simulink model "s_cd_hmc_reord_build_ramp"  (R2016b)
settings: Solver=VariableStepAuto  StartTime=0.0  StopTime=1000  RelTol=1e-3  EnableMultiTasking=on
undefined symbols (not defined in the file): Down, fft_stages, Up
libraries: xbsIndex_r4 x4695, casper_library_misc x3
(part 7 of 31)

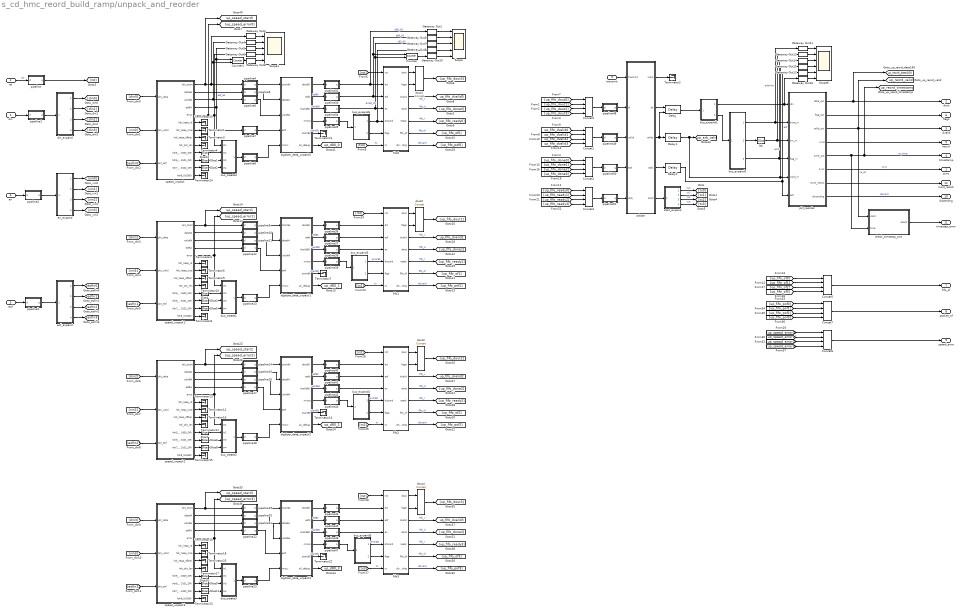
== system s_cd_hmc_reord_build_ramp/unpack_and_reorder ==
  rst : Inport
  din : Inport  Port=2
  eof : Inport  Port=3
  en : Inport  Port=4
  transmit : Inport  Port=5
  Concat{1..7} (7 alike) : xbsIndex_r4/Concat  num_inputs=4  dbl_ovrd=off  block_type=concat
  Counter : xbsIndex_r4/Counter  cnt_type=Free Running  cnt_to=Inf  operation=Up  start_count=0  cnt_by_val=1  arith_type=Unsigned  n_bits=10  bin_pt=0  load_pin=off  rst=on  en=on  explicit_period=on  period=1  use_behavioral_HDL=on  implementation=Fabric  dbl_ovrd=off  block_type=counter
  Counter1 : xbsIndex_r4/Counter  cnt_type=Free Running  cnt_to=Inf  operation=Up  start_count=0  cnt_by_val=1  arith_type=Unsigned  n_bits=10  bin_pt=0  load_pin=off  rst=on  en=on  explicit_period=on  period=1  use_behavioral_HDL=on  implementation=Fabric  dbl_ovrd=off  block_type=counter
  Delay : xbsIndex_r4/Delay  rst=off  infoeditControl=Selection of Reset will increase slice count due to use of real FFs and instead of SRLs  en=on  latency=1  reg_retiming=on  dbl_ovrd=off  block_type=delay
  Delay1 : xbsIndex_r4/Delay  rst=off  infoeditControl=Selection of Reset will increase slice count due to use of real FFs and instead of SRLs  en=off  latency=1  reg_retiming=on  dbl_ovrd=off  block_type=delay
  Delay2 : xbsIndex_r4/Delay  rst=off  infoeditControl=Selection of Reset will increase slice count due to use of real FFs and instead of SRLs  en=off  latency=1  reg_retiming=on  dbl_ovrd=off  block_type=delay
  Gateway Out{1..16} (16 alike) : xbsIndex_r4/Gateway Out  inherit_from_input=off  hdl_port=off  rows=1  columns=1  UseAsDAC=off  DACChannel='1'  interface=None  automatic_assignment=on  address_offset=hex2dec('00')  intf_name=''  intf_description=''  timing_constraint=None  locs_specified=off  LOCs={}  io_standard={}  block_type=gatewayout
  Scope : Scope  NumInputPorts=5
  Scope1 : Scope  NumInputPorts=5
  Scope6 : Scope  NumInputPorts=6
  Slice{1..3,5..6,8..9,11} (8 alike) : xbsIndex_r4/Slice  nbits=2  boolean_output=off  mode=Lower Bit Location + Width  bit1=0  base1=MSB of Input  bit0=0  base0=LSB of Input  dbl_ovrd=off  block_type=slice
  Slice{4,7,10,12} (4 alike) : xbsIndex_r4/Slice  nbits=48 - n_bits_timestep  boolean_output=off  mode=Upper Bit Location + Width  bit1=0  base1=MSB of Input  bit0=0  base0=LSB of Input  dbl_ovrd=off  block_type=slice
  Terminator{1..25} (25 alike) : Terminator
  arbiter : Subsystem  mask{n_inputs=4, n_bits_input=160 + 48 - n_bits_timestep + 2 + 2, mux_latency=2}
      mask prompts: n_inputs "number of inputs"; n_bits_input "input bit widths"; mux_latency "mux latency"
      mask init:
      | set_param([gcb, '/eofi_mux'], ...
      |     'n_bits', 'ones(1, n_inputs)', ...
      |     'mux_latency', 'mux_latency', ...
      |     'cmplx', 'off', 'misc', 'off');
      | set_param([gcb, '/di_mux'], ...
      |     'n_bits', 'repmat(n_bits_input, 1, n_inputs)', ...
      |     'mux_latency', 'mux_latency', ...
      |     'cmplx', 'off', 'misc', 'off');
      | set_param([gcb, '/validi_mux'], ...
      |     'n_bits', 'ones(1, n_inputs)', ...
      |     'mux_latency', 'mux_latency', ...
      |     'cmplx', 'off', 'misc', 'off');
      | set_param([gcb, '/busy_edge_rep'], ...
      |     'replication', 'n_inputs', ...
      |     'misc', 'off');
  bus_create1 : Subsystem  AncestorBlock=casper_library_flow_control/bus_create  mask(bus_create){inputNum=4}
      mask prompts: inputNum "Number of inputs:"
      mask init:
      | bus_create_init(gcb,...
      |     'inputNum', inputNum);
  bus_create2 : Subsystem  AncestorBlock=casper_library_flow_control/bus_create  mask(bus_create){inputNum=4}
      mask prompts: inputNum "Number of inputs:"
      mask init:
      | bus_create_init(gcb,...
      |     'inputNum', inputNum);
  bus_create3 : Subsystem  AncestorBlock=casper_library_flow_control/bus_create  mask(bus_create){inputNum=4}
      mask prompts: inputNum "Number of inputs:"
      mask init:
      | bus_create_init(gcb,...
      |     'inputNum', inputNum);
  bus_create4 : Subsystem  AncestorBlock=casper_library_flow_control/bus_create  mask(bus_create){inputNum=4}
      mask prompts: inputNum "Number of inputs:"
      mask init:
      | bus_create_init(gcb,...
      |     'inputNum', inputNum);
  bus_expand1 : Subsystem  AncestorBlock=casper_library_flow_control/bus_expand  mask(bus_expand){mode=divisions of arbitrary size, outputNum=1, outputWidth=[160, sum([48 - n_bits_timestep, 2, 2])], outputBinaryPt=[0 0], outputArithmeticType=[0 0], show_format=off, outputToWorkspace=off, variablePrefix=out, outputToModelAsWell=on}
      mask prompts: outputNum "Number of outputs:"; outputWidth "Output width [msb ... lsb]:"; outputBinaryPt "Output binary point position [msb ... lsb]:"; outputArithmeticType "Output arithmetic type (ufix=0, fix=1, bool=2) [msb ... lsb]:"; show_format "Print format string?"; outputToWorkspace "Output to workspace?"; variablePrefix "Variable name prefix:"; outputToModelAsWell "Output to model as well?"
      mask help:
      | Expands a 'bus' made using a bus_create or Xilinx
      | concat block.
      | The input will be divided into the specified number
      | of outputs with the specified arithmetic types.
      | Divisions are made from most significant bit.
      mask init: same as s_cd_hmc_reord_build_ramp/bus_expand
      settings: AttributesFormatString=2 outputs
      mask TypeOptions mode: divisions of equal size | divisions of arbitrary size
      mask Callback mode: bus_expand_callback();
      mask Callback outputWidth: bus_expand_callback();
      mask Callback outputToWorkspace: bus_expand_callback();
  bus_expand2 : Subsystem  AncestorBlock=casper_library_flow_control/bus_expand  mask(bus_expand){mode=divisions of arbitrary size, outputNum=1, outputWidth=[48 - n_bits_timestep, 2, 2], outputBinaryPt=[0 0 0], outputArithmeticType=[0 0 0], show_format=off, outputToWorkspace=off, variablePrefix=out, outputToModelAsWell=on}
      mask prompts: outputNum "Number of outputs:"; outputWidth "Output width [msb ... lsb]:"; outputBinaryPt "Output binary point position [msb ... lsb]:"; outputArithmeticType "Output arithmetic type (ufix=0, fix=1, bool=2) [msb ... lsb]:"; show_format "Print format string?"; outputToWorkspace "Output to workspace?"; variablePrefix "Variable name prefix:"; outputToModelAsWell "Output to model as well?"
      mask help:
      | Expands a 'bus' made using a bus_create or Xilinx
      | concat block.
      | The input will be divided into the specified number
      | of outputs with the specified arithmetic types.
      | Divisions are made from most significant bit.
      mask init: same as s_cd_hmc_reord_build_ramp/bus_expand
      settings: AttributesFormatString=3 outputs
      mask TypeOptions mode: divisions of equal size | divisions of arbitrary size
      mask Callback mode: bus_expand_callback();
      mask Callback outputWidth: bus_expand_callback();
      mask Callback outputToWorkspace: bus_expand_callback();
  bus_expand3 : Subsystem  AncestorBlock=casper_library_flow_control/bus_expand  mask(bus_expand){mode=divisions of arbitrary size, outputNum=1, outputWidth=[1, sum([48 - n_bits_timestep, 2, 2])], outputBinaryPt=[0 0], outputArithmeticType=[2 0], show_format=off, outputToWorkspace=off, variablePrefix=out, outputToModelAsWell=on}
      mask prompts: outputNum "Number of outputs:"; outputWidth "Output width [msb ... lsb]:"; outputBinaryPt "Output binary point position [msb ... lsb]:"; outputArithmeticType "Output arithmetic type (ufix=0, fix=1, bool=2) [msb ... lsb]:"; show_format "Print format string?"; outputToWorkspace "Output to workspace?"; variablePrefix "Variable name prefix:"; outputToModelAsWell "Output to model as well?"
      mask help:
      | Expands a 'bus' made using a bus_create or Xilinx
      | concat block.
      | The input will be divided into the specified number
      | of outputs with the specified arithmetic types.
      | Divisions are made from most significant bit.
      mask init: same as s_cd_hmc_reord_build_ramp/bus_expand
      settings: AttributesFormatString=2 outputs
      mask TypeOptions mode: divisions of equal size | divisions of arbitrary size
      mask Callback mode: bus_expand_callback();
      mask Callback outputWidth: bus_expand_callback();
      mask Callback outputToWorkspace: bus_expand_callback();
  bus_expand4 : Subsystem  AncestorBlock=casper_library_flow_control/bus_expand  mask(bus_expand){mode=divisions of arbitrary size, outputNum=1, outputWidth=[1, sum([48 - n_bits_timestep, 2, 2])], outputBinaryPt=[0 0], outputArithmeticType=[2 0], show_format=off, outputToWorkspace=off, variablePrefix=out, outputToModelAsWell=on}
      mask prompts: outputNum "Number of outputs:"; outputWidth "Output width [msb ... lsb]:"; outputBinaryPt "Output binary point position [msb ... lsb]:"; outputArithmeticType "Output arithmetic type (ufix=0, fix=1, bool=2) [msb ... lsb]:"; show_format "Print format string?"; outputToWorkspace "Output to workspace?"; variablePrefix "Variable name prefix:"; outputToModelAsWell "Output to model as well?"
      mask help:
      | Expands a 'bus' made using a bus_create or Xilinx
      | concat block.
      | The input will be divided into the specified number
      | of outputs with the specified arithmetic types.
      | Divisions are made from most significant bit.
      mask init: same as s_cd_hmc_reord_build_ramp/bus_expand
      settings: AttributesFormatString=2 outputs
      mask TypeOptions mode: divisions of equal size | divisions of arbitrary size
      mask Callback mode: bus_expand_callback();
      mask Callback outputWidth: bus_expand_callback();
      mask Callback outputToWorkspace: bus_expand_callback();
  bus_expand5 : Subsystem  AncestorBlock=casper_library_flow_control/bus_expand  mask(bus_expand){mode=divisions of arbitrary size, outputNum=1, outputWidth=[1, sum([48 - n_bits_timestep, 2, 2])], outputBinaryPt=[0 0], outputArithmeticType=[2 0], show_format=off, outputToWorkspace=off, variablePrefix=out, outputToModelAsWell=on}
      mask prompts: outputNum "Number of outputs:"; outputWidth "Output width [msb ... lsb]:"; outputBinaryPt "Output binary point position [msb ... lsb]:"; outputArithmeticType "Output arithmetic type (ufix=0, fix=1, bool=2) [msb ... lsb]:"; show_format "Print format string?"; outputToWorkspace "Output to workspace?"; variablePrefix "Variable name prefix:"; outputToModelAsWell "Output to model as well?"
      mask help:
      | Expands a 'bus' made using a bus_create or Xilinx
      | concat block.
      | The input will be divided into the specified number
      | of outputs with the specified arithmetic types.
      | Divisions are made from most significant bit.
      mask init: same as s_cd_hmc_reord_build_ramp/bus_expand
      settings: AttributesFormatString=2 outputs
      mask TypeOptions mode: divisions of equal size | divisions of arbitrary size
      mask Callback mode: bus_expand_callback();
      mask Callback outputWidth: bus_expand_callback();
      mask Callback outputToWorkspace: bus_expand_callback();
  bus_expand6 : Subsystem  AncestorBlock=casper_library_flow_control/bus_expand  mask(bus_expand){mode=divisions of arbitrary size, outputNum=1, outputWidth=[1, sum([48 - n_bits_timestep, 2, 2])], outputBinaryPt=[0 0], outputArithmeticType=[2 0], show_format=off, outputToWorkspace=off, variablePrefix=out, outputToModelAsWell=on}
      mask prompts: outputNum "Number of outputs:"; outputWidth "Output width [msb ... lsb]:"; outputBinaryPt "Output binary point position [msb ... lsb]:"; outputArithmeticType "Output arithmetic type (ufix=0, fix=1, bool=2) [msb ... lsb]:"; show_format "Print format string?"; outputToWorkspace "Output to workspace?"; variablePrefix "Variable name prefix:"; outputToModelAsWell "Output to model as well?"
      mask help:
      | Expands a 'bus' made using a bus_create or Xilinx
      | concat block.
      | The input will be divided into the specified number
      | of outputs with the specified arithmetic types.
      | Divisions are made from most significant bit.
      mask init: same as s_cd_hmc_reord_build_ramp/bus_expand
      settings: AttributesFormatString=2 outputs
      mask TypeOptions mode: divisions of equal size | divisions of arbitrary size
      mask Callback mode: bus_expand_callback();
      mask Callback outputWidth: bus_expand_callback();
      mask Callback outputToWorkspace: bus_expand_callback();
  check_timestep_one : Subsystem
  digitiser_data_unpack0 : Subsystem
  digitiser_data_unpack1 : Subsystem
  digitiser_data_unpack2 : Subsystem
  digitiser_data_unpack3 : Subsystem
  din_expand : Subsystem  AncestorBlock=casper_library_flow_control/bus_expand  mask(bus_expand){mode=divisions of equal size, outputNum=4, outputWidth=64, outputBinaryPt=0, outputArithmeticType=0, show_format=off, outputToWorkspace=off, variablePrefix=out, outputToModelAsWell=on}
      mask prompts: outputNum "Number of outputs:"; outputWidth "Output width:"; outputBinaryPt "Output binary point position:"; outputArithmeticType "Output arithmetic type (ufix=0, fix=1, bool=2):"; show_format "Print format string?"; outputToWorkspace "Output to workspace?"; variablePrefix "Variable name prefix:"; outputToModelAsWell "Output to model as well?"
      mask help:
      | Expands a 'bus' made using a bus_create or Xilinx
      | concat block.
      | The input will be divided into the specified number
      | of outputs with the specified arithmetic types.
      | Divisions are made from most significant bit.
      mask init: same as s_cd_hmc_reord_build_ramp/bus_expand
      settings: AttributesFormatString=4 outputs
      mask TypeOptions mode: divisions of equal size | divisions of arbitrary size
      mask Callback mode: bus_expand_callback();
      mask Callback outputWidth: bus_expand_callback();
      mask Callback outputToWorkspace: bus_expand_callback();
  dout{1..4} (4 alike) : xbsIndex_r4/Concat  num_inputs=2  dbl_ovrd=off  block_type=concat
  en_expand : Subsystem  AncestorBlock=casper_library_flow_control/bus_expand  mask(bus_expand){mode=divisions of equal size, outputNum=4, outputWidth=1, outputBinaryPt=0, outputArithmeticType=2, show_format=off, outputToWorkspace=off, variablePrefix=out, outputToModelAsWell=on}
      mask prompts: outputNum "Number of outputs:"; outputWidth "Output width:"; outputBinaryPt "Output binary point position:"; outputArithmeticType "Output arithmetic type (ufix=0, fix=1, bool=2):"; show_format "Print format string?"; outputToWorkspace "Output to workspace?"; variablePrefix "Variable name prefix:"; outputToModelAsWell "Output to model as well?"
      mask help:
      | Expands a 'bus' made using a bus_create or Xilinx
      | concat block.
      | The input will be divided into the specified number
      | of outputs with the specified arithmetic types.
      | Divisions are made from most significant bit.
      mask init: same as s_cd_hmc_reord_build_ramp/bus_expand
      settings: AttributesFormatString=4 outputs
      mask TypeOptions mode: divisions of equal size | divisions of arbitrary size
      mask Callback mode: bus_expand_callback();
      mask Callback outputWidth: bus_expand_callback();
      mask Callback outputToWorkspace: bus_expand_callback();
  eof_expand : Subsystem  AncestorBlock=casper_library_flow_control/bus_expand  mask(bus_expand){mode=divisions of equal size, outputNum=4, outputWidth=1, outputBinaryPt=0, outputArithmeticType=2, show_format=off, outputToWorkspace=off, variablePrefix=out, outputToModelAsWell=on}
      mask prompts: outputNum "Number of outputs:"; outputWidth "Output width:"; outputBinaryPt "Output binary point position:"; outputArithmeticType "Output arithmetic type (ufix=0, fix=1, bool=2):"; show_format "Print format string?"; outputToWorkspace "Output to workspace?"; variablePrefix "Variable name prefix:"; outputToModelAsWell "Output to model as well?"
      mask help:
      | Expands a 'bus' made using a bus_create or Xilinx
      | concat block.
      | The input will be divided into the specified number
      | of outputs with the specified arithmetic types.
      | Divisions are made from most significant bit.
      mask init: same as s_cd_hmc_reord_build_ramp/bus_expand
      settings: AttributesFormatString=4 outputs
      mask TypeOptions mode: divisions of equal size | divisions of arbitrary size
      mask Callback mode: bus_expand_callback();
      mask Callback outputWidth: bus_expand_callback();
      mask Callback outputToWorkspace: bus_expand_callback();
  fifo0 : Subsystem  mask{n_bits_din=80, scale_factor_bits=1, input_word_count_bits=n_bits_packet_size, n_bits_depth=n_bits_fifo_depth, n_bits_flag=sum([48 - n_bits_timestep, 2, 2]), bram_latency=bram_latency}
      mask prompts: n_bits_din "input data bit width"; scale_factor_bits "output width scale factor (2^? input bits)"; input_word_count_bits "max input word count (2^?)"; n_bits_depth "max buffer depth (2^? packets)"; n_bits_flag "flag bit width"; bram_latency "BRAM latency"
  fifo1 : Subsystem  mask{n_bits_din=80, scale_factor_bits=1, input_word_count_bits=n_bits_packet_size, n_bits_depth=n_bits_fifo_depth, n_bits_flag=sum([48 - n_bits_timestep, 2, 2]), bram_latency=bram_latency}
      mask prompts: n_bits_din "input data bit width"; scale_factor_bits "output width scale factor (2^? input bits)"; input_word_count_bits "max input word count (2^?)"; n_bits_depth "max buffer depth (2^? packets)"; n_bits_flag "flag bit width"; bram_latency "BRAM latency"
  fifo2 : Subsystem  mask{n_bits_din=80, scale_factor_bits=1, input_word_count_bits=n_bits_packet_size, n_bits_depth=n_bits_fifo_depth, n_bits_flag=sum([48 - n_bits_timestep, 2, 2]), bram_latency=bram_latency}
      mask prompts: n_bits_din "input data bit width"; scale_factor_bits "output width scale factor (2^? input bits)"; input_word_count_bits "max input word count (2^?)"; n_bits_depth "max buffer depth (2^? packets)"; n_bits_flag "flag bit width"; bram_latency "BRAM latency"
  fifo3 : Subsystem  mask{n_bits_din=80, scale_factor_bits=1, input_word_count_bits=n_bits_packet_size, n_bits_depth=n_bits_fifo_depth, n_bits_flag=sum([48 - n_bits_timestep, 2, 2]), bram_latency=bram_latency}
      mask prompts: n_bits_din "input data bit width"; scale_factor_bits "output width scale factor (2^? input bits)"; input_word_count_bits "max input word count (2^?)"; n_bits_depth "max buffer depth (2^? packets)"; n_bits_flag "flag bit width"; bram_latency "BRAM latency"
  lsb : xbsIndex_r4/Slice  nbits=1  boolean_output=off  mode=Lower Bit Location + Width  bit1=0  base1=MSB of Input  bit0=0  base0=LSB of Input  dbl_ovrd=off  block_type=slice
  pipeline : Subsystem  AncestorBlock=casper_library_delays/pipeline  mask(pipeline){latency=2}
      mask help:
      | An explicitly laid-out delay line to avoid mapping to SRL16s
      | for use in pipelining to help achieve timing closure.
      mask init:
      | pipeline_init(gcb,'latency',latency);
      settings: AttributesFormatString=Latency = %<latency>
      mask Display:
      | port_label('input', 1, 'd');
      | port_label('output', 1, 'q');
      | disp(['Z^-', num2str(latency)]);
  pipeline1 : Subsystem  AncestorBlock=casper_library_delays/pipeline  mask(pipeline){latency=2}
      mask help:
      | An explicitly laid-out delay line to avoid mapping to SRL16s
      | for use in pipelining to help achieve timing closure.
      mask init:
      | pipeline_init(gcb,'latency',latency);
      settings: AttributesFormatString=Latency = %<latency>
      mask Display:
      | port_label('input', 1, 'd');
      | port_label('output', 1, 'q');
      | disp(['Z^-', num2str(latency)]);
  pipeline10 : Subsystem  AncestorBlock=casper_library_delays/pipeline  mask(pipeline){latency=2}
      mask help:
      | An explicitly laid-out delay line to avoid mapping to SRL16s
      | for use in pipelining to help achieve timing closure.
      mask init:
      | pipeline_init(gcb,'latency',latency);
      settings: AttributesFormatString=Latency = %<latency>
      mask Display:
      | port_label('input', 1, 'd');
      | port_label('output', 1, 'q');
      | disp(['Z^-', num2str(latency)]);
  pipeline11 : Subsystem  AncestorBlock=casper_library_delays/pipeline  mask(pipeline){latency=2}
      mask help:
      | An explicitly laid-out delay line to avoid mapping to SRL16s
      | for use in pipelining to help achieve timing closure.
      mask init:
      | pipeline_init(gcb,'latency',latency);
      settings: AttributesFormatString=Latency = %<latency>
      mask Display:
      | port_label('input', 1, 'd');
      | port_label('output', 1, 'q');
      | disp(['Z^-', num2str(latency)]);
  pipeline12 : Subsystem  AncestorBlock=casper_library_delays/pipeline  mask(pipeline){latency=2}
      mask help:
      | An explicitly laid-out delay line to avoid mapping to SRL16s
      | for use in pipelining to help achieve timing closure.
      mask init:
      | pipeline_init(gcb,'latency',latency);
      settings: AttributesFormatString=Latency = %<latency>
      mask Display:
      | port_label('input', 1, 'd');
      | port_label('output', 1, 'q');
      | disp(['Z^-', num2str(latency)]);
  pipeline13 : Subsystem  AncestorBlock=casper_library_delays/pipeline  mask(pipeline){latency=2}
      mask help:
      | An explicitly laid-out delay line to avoid mapping to SRL16s
      | for use in pipelining to help achieve timing closure.
      mask init:
      | pipeline_init(gcb,'latency',latency);
      settings: AttributesFormatString=Latency = %<latency>
      mask Display:
      | port_label('input', 1, 'd');
      | port_label('output', 1, 'q');
      | disp(['Z^-', num2str(latency)]);
  pipeline14 : Subsystem  AncestorBlock=casper_library_delays/pipeline  mask(pipeline){latency=2}
      mask help:
      | An explicitly laid-out delay line to avoid mapping to SRL16s
      | for use in pipelining to help achieve timing closure.
      mask init:
      | pipeline_init(gcb,'latency',latency);
      settings: AttributesFormatString=Latency = %<latency>
      mask Display:
      | port_label('input', 1, 'd');
      | port_label('output', 1, 'q');
      | disp(['Z^-', num2str(latency)]);
  pipeline15 : Subsystem  AncestorBlock=casper_library_delays/pipeline  mask(pipeline){latency=2}
      mask help:
      | An explicitly laid-out delay line to avoid mapping to SRL16s
      | for use in pipelining to help achieve timing closure.
      mask init:
      | pipeline_init(gcb,'latency',latency);
      settings: AttributesFormatString=Latency = %<latency>
      mask Display:
      | port_label('input', 1, 'd');
      | port_label('output', 1, 'q');
      | disp(['Z^-', num2str(latency)]);
  pipeline16 : Subsystem  AncestorBlock=casper_library_delays/pipeline  mask(pipeline){latency=2}
      mask help:
      | An explicitly laid-out delay line to avoid mapping to SRL16s
      | for use in pipelining to help achieve timing closure.
      mask init:
      | pipeline_init(gcb,'latency',latency);
      settings: AttributesFormatString=Latency = %<latency>
      mask Display:
      | port_label('input', 1, 'd');
      | port_label('output', 1, 'q');
      | disp(['Z^-', num2str(latency)]);
  pipeline17 : Subsystem  AncestorBlock=casper_library_delays/pipeline  mask(pipeline){latency=2}
      mask help:
      | An explicitly laid-out delay line to avoid mapping to SRL16s
      | for use in pipelining to help achieve timing closure.
      mask init:
      | pipeline_init(gcb,'latency',latency);
      settings: AttributesFormatString=Latency = %<latency>
      mask Display:
      | port_label('input', 1, 'd');
      | port_label('output', 1, 'q');
      | disp(['Z^-', num2str(latency)]);
  pipeline18 : Subsystem  AncestorBlock=casper_library_delays/pipeline  mask(pipeline){latency=2}
      mask help:
      | An explicitly laid-out delay line to avoid mapping to SRL16s
      | for use in pipelining to help achieve timing closure.
      mask init:
      | pipeline_init(gcb,'latency',latency);
      settings: AttributesFormatString=Latency = %<latency>
      mask Display:
      | port_label('input', 1, 'd');
      | port_label('output', 1, 'q');
      | disp(['Z^-', num2str(latency)]);
  pipeline19 : Subsystem  AncestorBlock=casper_library_delays/pipeline  mask(pipeline){latency=2}
      mask help:
      | An explicitly laid-out delay line to avoid mapping to SRL16s
      | for use in pipelining to help achieve timing closure.
      mask init:
      | pipeline_init(gcb,'latency',latency);
      settings: AttributesFormatString=Latency = %<latency>
      mask Display:
      | port_label('input', 1, 'd');
      | port_label('output', 1, 'q');
      | disp(['Z^-', num2str(latency)]);
  pipeline2 : Subsystem  AncestorBlock=casper_library_delays/pipeline  mask(pipeline){latency=2}
      mask help:
      | An explicitly laid-out delay line to avoid mapping to SRL16s
      | for use in pipelining to help achieve timing closure.
      mask init:
      | pipeline_init(gcb,'latency',latency);
      settings: AttributesFormatString=Latency = %<latency>
      mask Display:
      | port_label('input', 1, 'd');
      | port_label('output', 1, 'q');
      | disp(['Z^-', num2str(latency)]);
  pipeline20 : Subsystem  AncestorBlock=casper_library_delays/pipeline  mask(pipeline){latency=2}
      mask help:
      | An explicitly laid-out delay line to avoid mapping to SRL16s
      | for use in pipelining to help achieve timing closure.
      mask init:
      | pipeline_init(gcb,'latency',latency);
      settings: AttributesFormatString=Latency = %<latency>
      mask Display:
      | port_label('input', 1, 'd');
      | port_label('output', 1, 'q');
      | disp(['Z^-', num2str(latency)]);
  pipeline21 : Subsystem  AncestorBlock=casper_library_delays/pipeline  mask(pipeline){latency=2}
      mask help:
      | An explicitly laid-out delay line to avoid mapping to SRL16s
      | for use in pipelining to help achieve timing closure.
      mask init:
      | pipeline_init(gcb,'latency',latency);
      settings: AttributesFormatString=Latency = %<latency>
      mask Display:
      | port_label('input', 1, 'd');
      | port_label('output', 1, 'q');
      | disp(['Z^-', num2str(latency)]);
  pipeline22 : Subsystem  AncestorBlock=casper_library_delays/pipeline  mask(pipeline){latency=2}
      mask help:
      | An explicitly laid-out delay line to avoid mapping to SRL16s
      | for use in pipelining to help achieve timing closure.
      mask init:
      | pipeline_init(gcb,'latency',latency);
      settings: AttributesFormatString=Latency = %<latency>
      mask Display:
      | port_label('input', 1, 'd');
      | port_label('output', 1, 'q');
      | disp(['Z^-', num2str(latency)]);
  pipeline23 : Subsystem  AncestorBlock=casper_library_delays/pipeline  mask(pipeline){latency=2}
      mask help:
      | An explicitly laid-out delay line to avoid mapping to SRL16s
      | for use in pipelining to help achieve timing closure.
      mask init:
      | pipeline_init(gcb,'latency',latency);
      settings: AttributesFormatString=Latency = %<latency>
      mask Display:
      | port_label('input', 1, 'd');
      | port_label('output', 1, 'q');
      | disp(['Z^-', num2str(latency)]);
  pipeline3 : Subsystem  AncestorBlock=casper_library_delays/pipeline  mask(pipeline){latency=2}
      mask help:
      | An explicitly laid-out delay line to avoid mapping to SRL16s
      | for use in pipelining to help achieve timing closure.
      mask init:
      | pipeline_init(gcb,'latency',latency);
      settings: AttributesFormatString=Latency = %<latency>
      mask Display:
      | port_label('input', 1, 'd');
      | port_label('output', 1, 'q');
      | disp(['Z^-', num2str(latency)]);
  pipeline32 : Subsystem  AncestorBlock=casper_library_delays/pipeline  mask(pipeline){latency=2}
      mask help:
      | An explicitly laid-out delay line to avoid mapping to SRL16s
      | for use in pipelining to help achieve timing closure.
      mask init:
      | pipeline_init(gcb,'latency',latency);
      settings: AttributesFormatString=Latency = %<latency>
      mask Display:
      | port_label('input', 1, 'd');
      | port_label('output', 1, 'q');
      | disp(['Z^-', num2str(latency)]);
  pipeline33 : Subsystem  AncestorBlock=casper_library_delays/pipeline  mask(pipeline){latency=2}
      mask help:
      | An explicitly laid-out delay line to avoid mapping to SRL16s
      | for use in pipelining to help achieve timing closure.
      mask init:
      | pipeline_init(gcb,'latency',latency);
      settings: AttributesFormatString=Latency = %<latency>
      mask Display:
      | port_label('input', 1, 'd');
      | port_label('output', 1, 'q');
      | disp(['Z^-', num2str(latency)]);
  pipeline34 : Subsystem  AncestorBlock=casper_library_delays/pipeline  mask(pipeline){latency=2}
      mask help:
      | An explicitly laid-out delay line to avoid mapping to SRL16s
      | for use in pipelining to help achieve timing closure.
      mask init:
      | pipeline_init(gcb,'latency',latency);
      settings: AttributesFormatString=Latency = %<latency>
      mask Display:
      | port_label('input', 1, 'd');
      | port_label('output', 1, 'q');
      | disp(['Z^-', num2str(latency)]);
  pipeline35 : Subsystem  AncestorBlock=casper_library_delays/pipeline  mask(pipeline){latency=2}
      mask help:
      | An explicitly laid-out delay line to avoid mapping to SRL16s
      | for use in pipelining to help achieve timing closure.
      mask init:
      | pipeline_init(gcb,'latency',latency);
      settings: AttributesFormatString=Latency = %<latency>
      mask Display:
      | port_label('input', 1, 'd');
      | port_label('output', 1, 'q');
      | disp(['Z^-', num2str(latency)]);
  pipeline36 : Subsystem  AncestorBlock=casper_library_delays/pipeline  mask(pipeline){latency=2}
      mask help:
      | An explicitly laid-out delay line to avoid mapping to SRL16s
      | for use in pipelining to help achieve timing closure.
      mask init:
      | pipeline_init(gcb,'latency',latency);
      settings: AttributesFormatString=Latency = %<latency>
      mask Display:
      | port_label('input', 1, 'd');
      | port_label('output', 1, 'q');
      | disp(['Z^-', num2str(latency)]);
  pipeline37 : Subsystem  AncestorBlock=casper_library_delays/pipeline  mask(pipeline){latency=2}
      mask help:
      | An explicitly laid-out delay line to avoid mapping to SRL16s
      | for use in pipelining to help achieve timing closure.
      mask init:
      | pipeline_init(gcb,'latency',latency);
      settings: AttributesFormatString=Latency = %<latency>
      mask Display:
      | port_label('input', 1, 'd');
      | port_label('output', 1, 'q');
      | disp(['Z^-', num2str(latency)]);
  pipeline38 : Subsystem  AncestorBlock=casper_library_delays/pipeline  mask(pipeline){latency=2}
      mask help:
      | An explicitly laid-out delay line to avoid mapping to SRL16s
      | for use in pipelining to help achieve timing closure.
      mask init:
      | pipeline_init(gcb,'latency',latency);
      settings: AttributesFormatString=Latency = %<latency>
      mask Display:
      | port_label('input', 1, 'd');
      | port_label('output', 1, 'q');
      | disp(['Z^-', num2str(latency)]);
  pipeline39 : Subsystem  AncestorBlock=casper_library_delays/pipeline  mask(pipeline){latency=2}
      mask help:
      | An explicitly laid-out delay line to avoid mapping to SRL16s
      | for use in pipelining to help achieve timing closure.
      mask init:
      | pipeline_init(gcb,'latency',latency);
      settings: AttributesFormatString=Latency = %<latency>
      mask Display:
      | port_label('input', 1, 'd');
      | port_label('output', 1, 'q');
      | disp(['Z^-', num2str(latency)]);
  pipeline4 : Subsystem  AncestorBlock=casper_library_delays/pipeline  mask(pipeline){latency=2}
      mask help:
      | An explicitly laid-out delay line to avoid mapping to SRL16s
      | for use in pipelining to help achieve timing closure.
      mask init:
      | pipeline_init(gcb,'latency',latency);
      settings: AttributesFormatString=Latency = %<latency>
      mask Display:
      | port_label('input', 1, 'd');
      | port_label('output', 1, 'q');
      | disp(['Z^-', num2str(latency)]);
  pipeline40 : Subsystem  AncestorBlock=casper_library_delays/pipeline  mask(pipeline){latency=2}
      mask help:
      | An explicitly laid-out delay line to avoid mapping to SRL16s
      | for use in pipelining to help achieve timing closure.
      mask init:
      | pipeline_init(gcb,'latency',latency);
      settings: AttributesFormatString=Latency = %<latency>
      mask Display:
      | port_label('input', 1, 'd');
      | port_label('output', 1, 'q');
      | disp(['Z^-', num2str(latency)]);
  pipeline41 : Subsystem  AncestorBlock=casper_library_delays/pipeline  mask(pipeline){latency=2}
      mask help:
      | An explicitly laid-out delay line to avoid mapping to SRL16s
      | for use in pipelining to help achieve timing closure.
      mask init:
      | pipeline_init(gcb,'latency',latency);
      settings: AttributesFormatString=Latency = %<latency>
      mask Display:
      | port_label('input', 1, 'd');
      | port_label('output', 1, 'q');
      | disp(['Z^-', num2str(latency)]);
  pipeline42 : Subsystem  AncestorBlock=casper_library_delays/pipeline  mask(pipeline){latency=2}
      mask help:
      | An explicitly laid-out delay line to avoid mapping to SRL16s
      | for use in pipelining to help achieve timing closure.
      mask init:
      | pipeline_init(gcb,'latency',latency);
      settings: AttributesFormatString=Latency = %<latency>
      mask Display:
      | port_label('input', 1, 'd');
      | port_label('output', 1, 'q');
      | disp(['Z^-', num2str(latency)]);
  pipeline43 : Subsystem  AncestorBlock=casper_library_delays/pipeline  mask(pipeline){latency=2}
      mask help:
      | An explicitly laid-out delay line to avoid mapping to SRL16s
      | for use in pipelining to help achieve timing closure.
      mask init:
      | pipeline_init(gcb,'latency',latency);
      settings: AttributesFormatString=Latency = %<latency>
      mask Display:
      | port_label('input', 1, 'd');
      | port_label('output', 1, 'q');
      | disp(['Z^-', num2str(latency)]);
  pipeline44 : Subsystem  AncestorBlock=casper_library_delays/pipeline  mask(pipeline){latency=2}
      mask help:
      | An explicitly laid-out delay line to avoid mapping to SRL16s
      | for use in pipelining to help achieve timing closure.
      mask init:
      | pipeline_init(gcb,'latency',latency);
      settings: AttributesFormatString=Latency = %<latency>
      mask Display:
      | port_label('input', 1, 'd');
      | port_label('output', 1, 'q');
      | disp(['Z^-', num2str(latency)]);
  pipeline45 : Subsystem  AncestorBlock=casper_library_delays/pipeline  mask(pipeline){latency=2}
      mask help:
      | An explicitly laid-out delay line to avoid mapping to SRL16s
      | for use in pipelining to help achieve timing closure.
      mask init:
      | pipeline_init(gcb,'latency',latency);
      settings: AttributesFormatString=Latency = %<latency>
      mask Display:
      | port_label('input', 1, 'd');
      | port_label('output', 1, 'q');
      | disp(['Z^-', num2str(latency)]);
  pipeline46 : Subsystem  AncestorBlock=casper_library_delays/pipeline  mask(pipeline){latency=2}
      mask help:
      | An explicitly laid-out delay line to avoid mapping to SRL16s
      | for use in pipelining to help achieve timing closure.
      mask init:
      | pipeline_init(gcb,'latency',latency);
      settings: AttributesFormatString=Latency = %<latency>
      mask Display:
      | port_label('input', 1, 'd');
      | port_label('output', 1, 'q');
      | disp(['Z^-', num2str(latency)]);
  pipeline47 : Subsystem  AncestorBlock=casper_library_delays/pipeline  mask(pipeline){latency=2}
      mask help:
      | An explicitly laid-out delay line to avoid mapping to SRL16s
      | for use in pipelining to help achieve timing closure.
      mask init:
      | pipeline_init(gcb,'latency',latency);
      settings: AttributesFormatString=Latency = %<latency>
      mask Display:
      | port_label('input', 1, 'd');
      | port_label('output', 1, 'q');
      | disp(['Z^-', num2str(latency)]);
  pipeline48 : Subsystem  AncestorBlock=casper_library_delays/pipeline  mask(pipeline){latency=2}
      mask help:
      | An explicitly laid-out delay line to avoid mapping to SRL16s
      | for use in pipelining to help achieve timing closure.
      mask init:
      | pipeline_init(gcb,'latency',latency);
      settings: AttributesFormatString=Latency = %<latency>
      mask Display:
      | port_label('input', 1, 'd');
      | port_label('output', 1, 'q');
      | disp(['Z^-', num2str(latency)]);
  pipeline49 : Subsystem  AncestorBlock=casper_library_delays/pipeline  mask(pipeline){latency=2}
      mask help:
      | An explicitly laid-out delay line to avoid mapping to SRL16s
      | for use in pipelining to help achieve timing closure.
      mask init:
      | pipeline_init(gcb,'latency',latency);
      settings: AttributesFormatString=Latency = %<latency>
      mask Display:
      | port_label('input', 1, 'd');
      | port_label('output', 1, 'q');
      | disp(['Z^-', num2str(latency)]);
  pipeline5 : Subsystem  AncestorBlock=casper_library_delays/pipeline  mask(pipeline){latency=2}
      mask help:
      | An explicitly laid-out delay line to avoid mapping to SRL16s
      | for use in pipelining to help achieve timing closure.
      mask init:
      | pipeline_init(gcb,'latency',latency);
      settings: AttributesFormatString=Latency = %<latency>
      mask Display:
      | port_label('input', 1, 'd');
      | port_label('output', 1, 'q');
      | disp(['Z^-', num2str(latency)]);
  pipeline50 : Subsystem  AncestorBlock=casper_library_delays/pipeline  mask(pipeline){latency=2}
      mask help:
      | An explicitly laid-out delay line to avoid mapping to SRL16s
      | for use in pipelining to help achieve timing closure.
      mask init:
      | pipeline_init(gcb,'latency',latency);
      settings: AttributesFormatString=Latency = %<latency>
      mask Display:
      | port_label('input', 1, 'd');
      | port_label('output', 1, 'q');
      | disp(['Z^-', num2str(latency)]);
  pipeline51 : Subsystem  AncestorBlock=casper_library_delays/pipeline  mask(pipeline){latency=2}
      mask help:
      | An explicitly laid-out delay line to avoid mapping to SRL16s
      | for use in pipelining to help achieve timing closure.
      mask init:
      | pipeline_init(gcb,'latency',latency);
      settings: AttributesFormatString=Latency = %<latency>
      mask Display:
      | port_label('input', 1, 'd');
      | port_label('output', 1, 'q');
      | disp(['Z^-', num2str(latency)]);
  pipeline6 : Subsystem  AncestorBlock=casper_library_delays/pipeline  mask(pipeline){latency=2}
      mask help:
      | An explicitly laid-out delay line to avoid mapping to SRL16s
      | for use in pipelining to help achieve timing closure.
      mask init:
      | pipeline_init(gcb,'latency',latency);
      settings: AttributesFormatString=Latency = %<latency>
      mask Display:
      | port_label('input', 1, 'd');
      | port_label('output', 1, 'q');
      | disp(['Z^-', num2str(latency)]);
  pipeline7 : Subsystem  AncestorBlock=casper_library_delays/pipeline  mask(pipeline){latency=2}
      mask help:
      | An explicitly laid-out delay line to avoid mapping to SRL16s
      | for use in pipelining to help achieve timing closure.
      mask init:
      | pipeline_init(gcb,'latency',latency);
      settings: AttributesFormatString=Latency = %<latency>
      mask Display:
      | port_label('input', 1, 'd');
      | port_label('output', 1, 'q');
      | disp(['Z^-', num2str(latency)]);
  pipeline8 : Subsystem  AncestorBlock=casper_library_delays/pipeline  mask(pipeline){latency=2}
      mask help:
      | An explicitly laid-out delay line to avoid mapping to SRL16s
      | for use in pipelining to help achieve timing closure.
      mask init:
      | pipeline_init(gcb,'latency',latency);
      settings: AttributesFormatString=Latency = %<latency>
      mask Display:
      | port_label('input', 1, 'd');
      | port_label('output', 1, 'q');
      | disp(['Z^-', num2str(latency)]);
  pipeline9 : Subsystem  AncestorBlock=casper_library_delays/pipeline  mask(pipeline){latency=2}
      mask help:
      | An explicitly laid-out delay line to avoid mapping to SRL16s
      | for use in pipelining to help achieve timing closure.
      mask init:
      | pipeline_init(gcb,'latency',latency);
      settings: AttributesFormatString=Latency = %<latency>
      mask Display:
      | port_label('input', 1, 'd');
      | port_label('output', 1, 'q');
      | disp(['Z^-', num2str(latency)]);
  pkt_reorder : Subsystem  mask{window_bits=n_bits_buffer_depth, window_size_bits=n_bits_packet_size - 1, n_bits_din=80, n_bits_flag=2, n_bits_timestamp=48 - n_bits_timestep}
      mask prompts: window_bits "Number of Windows to Buffer (2^?)"; window_size_bits "Window size (2^?)"; n_bits_din "Data bit width in"; n_bits_flag "Flag bit width in"; n_bits_timestamp "Timestamp bit width"
      mask init:
      | fmtstr = sprintf('Buffer space: 2^%i words', window_bits+window_size_bits);
      | set_param(gcb, 'AttributesFormatString', fmtstr);
      settings: AttributesFormatString=Buffer space: 2^12 words
  spead_unpack : Subsystem  Tag=casper:spead_unpack  AncestorBlock=casper_library_communications/spead_unpack  mask(spead_unpack_mask){max_pkt_len_bits=10, header_ids=0x1600, 0x3101, 0x3102, header_ind_ids=0x3300, spead_msw=64, spead_lsw=48, spead_version=4, combine_errors=on}
      mask prompts: max_pkt_len_bits "Max pkt length, 2^? 64-bit words"; header_ids "SPEAD direct header IDs (decimal)"; header_ind_ids "SPEAD indirect address IDs (decimal)"; spead_msw "SPEAD Flavour (MSw)"; spead_lsw "SPEAD Flavour (LSw)"; spead_version "SPEAD version"; combine_errors "Combine error flags"
      mask help: This block receives a 64-bit-word stream that contains a SPEAD stream. It checks the SPEAD headers are being correctly received. It presents the user with all headers on the first valid cycle of data along with a flag to indicate a header or packet-length error.
      mask init:
      | spead_unpack_init(gcb)
  spead_unpack1 : Subsystem  Tag=casper:spead_unpack  AncestorBlock=casper_library_communications/spead_unpack  mask(spead_unpack_mask){max_pkt_len_bits=10, header_ids=0x1600, 0x3101, 0x3102, header_ind_ids=0x3300, spead_msw=64, spead_lsw=48, spead_version=4, combine_errors=on}
      mask prompts: max_pkt_len_bits "Max pkt length, 2^? 64-bit words"; header_ids "SPEAD direct header IDs (decimal)"; header_ind_ids "SPEAD indirect address IDs (decimal)"; spead_msw "SPEAD Flavour (MSw)"; spead_lsw "SPEAD Flavour (LSw)"; spead_version "SPEAD version"; combine_errors "Combine error flags"
      mask help: This block receives a 64-bit-word stream that contains a SPEAD stream. It checks the SPEAD headers are being correctly received. It presents the user with all headers on the first valid cycle of data along with a flag to indicate a header or packet-length error.
      mask init:
      | spead_unpack_init(gcb)
  spead_unpack2 : Subsystem  Tag=casper:spead_unpack  AncestorBlock=casper_library_communications/spead_unpack  mask(spead_unpack_mask){max_pkt_len_bits=10, header_ids=0x1600, 0x3101, 0x3102, header_ind_ids=0x3300, spead_msw=64, spead_lsw=48, spead_version=4, combine_errors=on}
      mask prompts: max_pkt_len_bits "Max pkt length, 2^? 64-bit words"; header_ids "SPEAD direct header IDs (decimal)"; header_ind_ids "SPEAD indirect address IDs (decimal)"; spead_msw "SPEAD Flavour (MSw)"; spead_lsw "SPEAD Flavour (LSw)"; spead_version "SPEAD version"; combine_errors "Combine error flags"
      mask help: This block receives a 64-bit-word stream that contains a SPEAD stream. It checks the SPEAD headers are being correctly received. It presents the user with all headers on the first valid cycle of data along with a flag to indicate a header or packet-length error.
      mask init:
      | spead_unpack_init(gcb)
  spead_unpack3 : Subsystem  Tag=casper:spead_unpack  AncestorBlock=casper_library_communications/spead_unpack  mask(spead_unpack_mask){max_pkt_len_bits=10, header_ids=0x1600, 0x3101, 0x3102, header_ind_ids=0x3300, spead_msw=64, spead_lsw=48, spead_version=4, combine_errors=on}
      mask prompts: max_pkt_len_bits "Max pkt length, 2^? 64-bit words"; header_ids "SPEAD direct header IDs (decimal)"; header_ind_ids "SPEAD indirect address IDs (decimal)"; spead_msw "SPEAD Flavour (MSw)"; spead_lsw "SPEAD Flavour (LSw)"; spead_version "SPEAD version"; combine_errors "Combine error flags"
      mask help: This block receives a 64-bit-word stream that contains a SPEAD stream. It checks the SPEAD headers are being correctly received. It presents the user with all headers on the first valid cycle of data along with a flag to indicate a header or packet-length error.
      mask init:
      | spead_unpack_init(gcb)
  start_expand : Subsystem  AncestorBlock=casper_library_flow_control/bus_expand  mask(bus_expand){mode=divisions of equal size, outputNum=4, outputWidth=1, outputBinaryPt=0, outputArithmeticType=2, show_format=off, outputToWorkspace=off, variablePrefix=out, outputToModelAsWell=on}
      mask prompts: outputNum "Number of outputs:"; outputWidth "Output width:"; outputBinaryPt "Output binary point position:"; outputArithmeticType "Output arithmetic type (ufix=0, fix=1, bool=2):"; show_format "Print format string?"; outputToWorkspace "Output to workspace?"; variablePrefix "Variable name prefix:"; outputToModelAsWell "Output to model as well?"
      mask help:
      | Expands a 'bus' made using a bus_create or Xilinx
      | concat block.
      | The input will be divided into the specified number
      | of outputs with the specified arithmetic types.
      | Divisions are made from most significant bit.
      mask init: same as s_cd_hmc_reord_build_ramp/bus_expand
      settings: AttributesFormatString=4 outputs
      mask TypeOptions mode: divisions of equal size | divisions of arbitrary size
      mask Callback mode: bus_expand_callback();
      mask Callback outputWidth: bus_expand_callback();
      mask Callback outputToWorkspace: bus_expand_callback();
  sync : Outport
  dout : Outport  Port=2
  dvalid : Outport  Port=3
  timestamp : Outport  Port=4
  recvd : Outport  Port=5
  flags : Outport  Port=6
  fifo_of : Outport  Port=7
  packet_of : Outport  Port=8
  spead_error : Outport  Port=9
  discarding : Outport  Port=10
  timestep_error : Outport  Port=11
  mcnt_relock : Outport  Port=12
  tag scope: up_arb_valid=global, up_d80_0=global, up_d80_1=global, up_d80_2=global, up_d80_3=global, up_fifo_dvalid0=global, up_fifo_dvalid1=global, up_fifo_dvalid2=global, up_fifo_dvalid3=global, up_reord_data160=global, up_reord_timestamp=global, up_reord_valid=global, up_spead_start0=global, up_spead_start1=global, up_spead_start2=global, up_spead_start3=global
  wires:
  digitiser_data_unpack0/6(all_debug) -> [up_d80_0]
  digitiser_data_unpack0/5(start80) -> Terminator21/1  "start80"
  spead_unpack/1(pkt_start) -> pipeline4/1(d), Gateway Out3/1, [up_spead_start0]
  [rst] -> fifo0/1(rst)
  Slice1/1 -> bus_create4/3(in3)
  Slice2/1 -> bus_create4/4(in4)
  Slice12/1 -> bus_create4/2(in2)
  spead_unpack/10(hdr5_0x1600_DIR) -> Slice12/1
  spead_unpack/11(hdr6_0x3101_DIR) -> Slice1/1
  spead_unpack/12(hdr7_0x3102_DIR) -> Slice2/1
  [tx0] -> fifo0/7(tx)  "tx"
  bus_expand6/2(lsb_out1) -> fifo0/6(flagi)
  digitiser_data_unpack0/4(misco) -> pipeline35/1(d)
  digitiser_data_unpack0/1(dout80) -> pipeline32/1(d)
  digitiser_data_unpack0/2(eofo) -> pipeline33/1(d)  "eof80"
  digitiser_data_unpack0/3(dvalid80) -> pipeline34/1(d)  "valid80"
  spead_unpack/6(hdr_heap_id) -> Terminator20/1
  spead_unpack/7(hdr_heap_size) -> Terminator1/1
  spead_unpack/8(hdr_heap_offset) -> Terminator3/1
  spead_unpack/9(hdr_pkt_len) -> Terminator4/1
  pkt_reorder/6(sync) -> sync/1  "sync"
  fifo0/4(done) -> [up_fifo_done0]  "fifo_d"
  dout1/1 -> [up_fifo_dout0]
  fifo0/3(dvalid) -> [up_fifo_dvalid0]  "fifo_v"
  fifo0/5(ready) -> [up_fifo_ready0]  "fifo_r"
  fifo0/6(fifo_of) -> [up_fifo_of0]  "fifo_of"
  arbiter/5(start) -> start_expand/1(bus_in)
  Concat4/1 -> pipeline51/1(d)
  Concat2/1 -> pipeline50/1(d)
  Concat3/1 -> pipeline48/1(d)
  Concat1/1 -> pipeline49/1(d)
  transmit/1 -> arbiter/1(transmit)
  start_expand/1(msb_out4) -> [tx0]  "tx0"
  start_expand/2(out3) -> [tx1]  "tx1"
  start_expand/3(out2) -> [tx2]  "tx2"
  start_expand/4(lsb_out1) -> [tx3]  "tx3"
  [up_fifo_done0] -> Concat2/1
  [up_fifo_done3] -> Concat2/4
  [up_fifo_done1] -> Concat2/2
  [up_fifo_done2] -> Concat2/3
  [up_fifo_dout0] -> Concat3/1
  [up_fifo_dout1] -> Concat3/2
  [up_fifo_dvalid0] -> Concat1/1
  [up_fifo_dvalid1] -> Concat1/2
  [up_fifo_ready0] -> Concat4/1
  [up_fifo_ready1] -> Concat4/2
  [up_fifo_dout2] -> Concat3/3
  [up_fifo_dout3] -> Concat3/4
  [up_fifo_dvalid2] -> Concat1/3
  [up_fifo_dvalid3] -> Concat1/4
  [up_fifo_ready2] -> Concat4/3
  [up_fifo_ready3] -> Concat4/4
  arbiter/1(input) -> Terminator2/1
  [up_fifo_of0] -> Concat5/1
  [up_fifo_of1] -> Concat5/2
  [up_fifo_of2] -> Concat5/3
  [up_fifo_of3] -> Concat5/4
  rst/1 -> pipeline/1(d)  "rst"
  din/1 -> pipeline1/1(d)
  en/1 -> pipeline2/1(d)
  eof/1 -> pipeline3/1(d)
  bus_expand1/2(lsb_out1) -> bus_expand2/1(bus_in)
  bus_expand2/1(msb_out3) -> Gateway Out11/1, pkt_reorder/2(time_in)  "arbtime"
  fifo0/1(dout) -> dout1/1
  fifo0/2(flago) -> dout1/2
  bus_expand2/2(out2) -> lsb/1
  arbiter/2(do) -> Delay/1
  arbiter/3(valido) -> Delay1/1, Delay/2
  arbiter/4(eofo) -> Delay2/1
  Delay/1 -> bus_expand1/1(bus_in)
  Delay1/1 -> Gateway Out15/1, pkt_reorder/5(valid_in), [up_arb_valid]  "valid"
  Delay2/1 -> pkt_reorder/6(eof), Gateway Out12/1  "eof"
  [up_spead_error0] -> Concat6/1
  [up_spead_error1] -> Concat6/2
  [up_spead_error2] -> Concat6/3
  [up_spead_error3] -> Concat6/4
  fifo0/7(discading) -> [up_fifo_pof0]  "discard"
  [up_fifo_pof0] -> Concat7/1
  [up_fifo_pof1] -> Concat7/2
  [up_fifo_pof2] -> Concat7/3
  [up_fifo_pof3] -> Concat7/4
  pkt_reorder/8(discarding) -> discarding/1  "discard"
  pkt_reorder/5(time_out) -> check_timestep_one/2(time), [up_reord_timestamp], timestamp/1  "re_time"
  pkt_reorder/3(valid_out) -> dvalid/1, check_timestep_one/1(valid), [up_reord_valid]  "re_en"
  spead_unpack/13(hdr8_0x3300) -> Terminator24/1
  din_expand/1(msb_out4) -> [din0]
  din_expand/2(out3) -> [din1]
  din_expand/3(out2) -> [din2]
  din_expand/4(lsb_out1) -> [din3]
  [din0] -> spead_unpack/1(pkt_data)
  en_expand/1(msb_out4) -> [vin0]
  en_expand/2(out3) -> [vin1]
  en_expand/3(out2) -> [vin2]
  en_expand/4(lsb_out1) -> [vin3]
  eof_expand/1(msb_out4) -> [eofin0]
  eof_expand/2(out3) -> [eofin1]
  eof_expand/3(out2) -> [eofin2]
  eof_expand/4(lsb_out1) -> [eofin3]
  [vin0] -> spead_unpack/2(pkt_valid)
  [eofin0] -> spead_unpack/3(pkt_eof)
  digitiser_data_unpack1/6(all_debug) -> [up_d80_1]
  digitiser_data_unpack1/5(start80) -> Terminator7/1  "start80"
  spead_unpack1/5(error) -> bus_create1/1(in1), [up_spead_error1]
  [rst] -> fifo1/1(rst)
  Slice3/1 -> bus_create1/3(in3)
  Slice5/1 -> bus_create1/4(in4)
  Slice4/1 -> bus_create1/2(in2)
  spead_unpack1/10(hdr5_0x1600_DIR) -> Slice4/1
  spead_unpack1/11(hdr6_0x3101_DIR) -> Slice3/1
  spead_unpack1/12(hdr7_0x3102_DIR) -> Slice5/1
  [tx1] -> fifo1/7(tx)  "tx"
  bus_expand3/1(msb_out2) -> fifo1/5(discard)  "error80"
  bus_expand3/2(lsb_out1) -> fifo1/6(flagi)
  digitiser_data_unpack1/4(misco) -> pipeline39/1(d)
  digitiser_data_unpack1/1(dout80) -> pipeline36/1(d)
  digitiser_data_unpack1/2(eofo) -> pipeline37/1(d)  "eof80"
  digitiser_data_unpack1/3(dvalid80) -> pipeline38/1(d)  "valid80"
  spead_unpack1/6(hdr_heap_id) -> Terminator6/1
  spead_unpack1/7(hdr_heap_size) -> Terminator5/1
  spead_unpack1/8(hdr_heap_offset) -> Terminator9/1
  spead_unpack1/9(hdr_pkt_len) -> Terminator10/1
  fifo1/4(done) -> [up_fifo_done1]  "fifo_d"
  dout2/1 -> [up_fifo_dout1]
  fifo1/3(dvalid) -> [up_fifo_dvalid1]  "fifo_v"
  fifo1/5(ready) -> [up_fifo_ready1]  "fifo_r"
  fifo1/6(fifo_of) -> [up_fifo_of1]  "fifo_of"
  fifo1/1(dout) -> dout2/1
  fifo1/2(flago) -> dout2/2
  fifo1/7(discading) -> [up_fifo_pof1]  "discard"
  spead_unpack1/13(hdr8_0x3300) -> Terminator8/1
  [din1] -> spead_unpack1/1(pkt_data)
  [vin1] -> spead_unpack1/2(pkt_valid)
  [eofin1] -> spead_unpack1/3(pkt_eof)
  digitiser_data_unpack2/6(all_debug) -> [up_d80_2]
  digitiser_data_unpack2/5(start80) -> Terminator14/1  "start80"
  spead_unpack2/5(error) -> [up_spead_error2], bus_create2/1(in1)
  [rst] -> fifo2/1(rst)
  Slice6/1 -> bus_create2/3(in3)
  Slice8/1 -> bus_create2/4(in4)
  Slice7/1 -> bus_create2/2(in2)
  spead_unpack2/10(hdr5_0x1600_DIR) -> Slice7/1
  spead_unpack2/11(hdr6_0x3101_DIR) -> Slice6/1
  spead_unpack2/12(hdr7_0x3102_DIR) -> Slice8/1
  [tx2] -> fifo2/7(tx)  "tx"
  bus_expand4/1(msb_out2) -> fifo2/5(discard)  "error80"
  bus_expand4/2(lsb_out1) -> fifo2/6(flagi)
  digitiser_data_unpack2/4(misco) -> pipeline43/1(d)
  digitiser_data_unpack2/1(dout80) -> pipeline40/1(d)
  digitiser_data_unpack2/2(eofo) -> pipeline41/1(d)  "eof80"
  digitiser_data_unpack2/3(dvalid80) -> pipeline42/1(d)  "valid80"
  spead_unpack2/6(hdr_heap_id) -> Terminator13/1
  spead_unpack2/7(hdr_heap_size) -> Terminator12/1
  spead_unpack2/8(hdr_heap_offset) -> Terminator16/1
  spead_unpack2/9(hdr_pkt_len) -> Terminator11/1
  fifo2/4(done) -> [up_fifo_done2]  "fifo_d"
  dout3/1 -> [up_fifo_dout2]
  fifo2/3(dvalid) -> [up_fifo_dvalid2]  "fifo_v"
  fifo2/5(ready) -> [up_fifo_ready2]  "fifo_r"
  fifo2/6(fifo_of) -> [up_fifo_of2]  "fifo_of"
  fifo2/1(dout) -> dout3/1
  fifo2/2(flago) -> dout3/2
  fifo2/7(discading) -> [up_fifo_pof2]  "discard"
  spead_unpack2/13(hdr8_0x3300) -> Terminator15/1
  [din2] -> spead_unpack2/1(pkt_data)
  [vin2] -> spead_unpack2/2(pkt_valid)
  [eofin2] -> spead_unpack2/3(pkt_eof)
  digitiser_data_unpack3/6(all_debug) -> [up_d80_3]
  digitiser_data_unpack3/5(start80) -> Terminator22/1  "start80"
  spead_unpack3/5(error) -> bus_create3/1(in1), [up_spead_error3]
  [rst] -> fifo3/1(rst)
  Slice9/1 -> bus_create3/3(in3)
  Slice11/1 -> bus_create3/4(in4)
  Slice10/1 -> bus_create3/2(in2)
  spead_unpack3/10(hdr5_0x1600_DIR) -> Slice10/1
  spead_unpack3/11(hdr6_0x3101_DIR) -> Slice9/1
  spead_unpack3/12(hdr7_0x3102_DIR) -> Slice11/1
  [tx3] -> fifo3/7(tx)  "tx"
  bus_expand5/1(msb_out2) -> fifo3/5(discard)  "error80"
  bus_expand5/2(lsb_out1) -> fifo3/6(flagi)
  digitiser_data_unpack3/4(misco) -> pipeline47/1(d)
  digitiser_data_unpack3/1(dout80) -> pipeline44/1(d)
  digitiser_data_unpack3/2(eofo) -> pipeline45/1(d)  "eof80"
  digitiser_data_unpack3/3(dvalid80) -> pipeline46/1(d)  "valid80"
  spead_unpack3/6(hdr_heap_id) -> Terminator19/1
  spead_unpack3/7(hdr_heap_size) -> Terminator18/1
  spead_unpack3/8(hdr_heap_offset) -> Terminator25/1
  spead_unpack3/9(hdr_pkt_len) -> Terminator17/1
  fifo3/4(done) -> [up_fifo_done3]  "fifo_d"
  dout4/1 -> [up_fifo_dout3]
  fifo3/3(dvalid) -> [up_fifo_dvalid3]  "fifo_v"
  fifo3/5(ready) -> [up_fifo_ready3]  "fifo_r"
  fifo3/6(fifo_of) -> [up_fifo_of3]  "fifo_of"
  fifo3/1(dout) -> dout4/1
  fifo3/2(flago) -> dout4/2
  fifo3/7(discading) -> [up_fifo_pof3]  "discard"
  spead_unpack3/13(hdr8_0x3300) -> Terminator23/1
  [din3] -> spead_unpack3/1(pkt_data)
  [vin3] -> spead_unpack3/2(pkt_valid)
  [eofin3] -> spead_unpack3/3(pkt_eof)
  pkt_reorder/1(data_out) -> dout/1, [up_reord_data160]
  pkt_reorder/2(flag_out) -> flags/1
  pkt_reorder/4(rcvd) -> recvd/1
  check_timestep_one/1(relock) -> timestep_error/1
  pkt_reorder/7(mcnt_relock) -> mcnt_relock/1
  pipeline/1(q) -> [rst]
  pipeline1/1(q) -> din_expand/1(bus_in)
  pipeline2/1(q) -> en_expand/1(bus_in)
  pipeline3/1(q) -> eof_expand/1(bus_in)
  spead_unpack/2(data64) -> pipeline5/1(d)
  spead_unpack/3(valid64) -> pipeline6/1(d), Gateway Out4/1, Counter1/2
  bus_create4/1(bus_out) -> pipeline8/1(d)
  spead_unpack1/4(eof64) -> pipeline12/1(d)
  bus_create1/1(bus_out) -> pipeline13/1(d)
  spead_unpack1/3(valid64) -> pipeline11/1(d)
  spead_unpack1/2(data64) -> pipeline10/1(d)
  spead_unpack1/1(pkt_start) -> pipeline9/1(d), [up_spead_start1]
  bus_create2/1(bus_out) -> pipeline18/1(d)
  spead_unpack2/2(data64) -> pipeline15/1(d)
  spead_unpack2/3(valid64) -> pipeline16/1(d)
  spead_unpack2/1(pkt_start) -> pipeline14/1(d), [up_spead_start2]
  spead_unpack2/4(eof64) -> pipeline17/1(d)
  spead_unpack3/3(valid64) -> pipeline21/1(d)
  bus_create3/1(bus_out) -> pipeline23/1(d)
  spead_unpack3/2(data64) -> pipeline20/1(d)
  spead_unpack3/4(eof64) -> pipeline22/1(d)
  spead_unpack3/1(pkt_start) -> pipeline19/1(d), [up_spead_start3]
  pipeline35/1(q) -> bus_expand6/1(bus_in)
  pipeline36/1(q) -> fifo1/2(din)
  pipeline37/1(q) -> fifo1/3(eof)
  pipeline38/1(q) -> fifo1/4(en)
  pipeline39/1(q) -> bus_expand3/1(bus_in)
  pipeline40/1(q) -> fifo2/2(din)
  pipeline41/1(q) -> fifo2/3(eof)
  pipeline42/1(q) -> fifo2/4(en)
  pipeline43/1(q) -> bus_expand4/1(bus_in)
  pipeline44/1(q) -> fifo3/2(din)
  pipeline45/1(q) -> fifo3/3(eof)
  pipeline46/1(q) -> fifo3/4(en)
  pipeline47/1(q) -> bus_expand5/1(bus_in)
  pipeline48/1(q) -> arbiter/2(di)
  pipeline49/1(q) -> arbiter/3(validi)
  pipeline50/1(q) -> arbiter/4(eofi)
  pipeline51/1(q) -> arbiter/5(drdy)
  Concat6/1 -> spead_error/1
  Concat7/1 -> packet_of/1
  Concat5/1 -> fifo_of/1
  bus_expand1/1(msb_out2) -> Gateway Out16/1, pkt_reorder/1(din)
  bus_expand2/3(lsb_out1) -> Gateway Out14/1, pkt_reorder/4(flag_in)
  lsb/1 -> Gateway Out13/1, pkt_reorder/3(src_in)
  Gateway Out11/1 -> Scope6/1
  Gateway Out13/1 -> Scope6/2
  Gateway Out14/1 -> Scope6/3
  Gateway Out15/1 -> Scope6/4
  Gateway Out12/1 -> Scope6/5
  Gateway Out16/1 -> Scope6/6
  pipeline32/1(q) -> fifo0/2(din), Gateway Out1/1  "d80_00"
  pipeline33/1(q) -> fifo0/3(eof), Gateway Out2/1, Counter/1  "e80_00"
  pipeline34/1(q) -> fifo0/4(en), Gateway Out7/1, Counter/2  "v80_00"
  bus_expand6/1(msb_out2) -> fifo0/5(discard), Gateway Out9/1  "err80_00"
  Gateway Out1/1 -> Scope/1
  Gateway Out2/1 -> Scope/2
  Gateway Out7/1 -> Scope/3
  Gateway Out9/1 -> Scope/4
  Counter/1 -> Gateway Out10/1
  Gateway Out10/1 -> Scope/5
  spead_unpack/4(eof64) -> pipeline7/1(d), Gateway Out5/1, Counter1/1  "eof_64"
  Gateway Out3/1 -> Scope1/1
  Gateway Out4/1 -> Scope1/2
  Gateway Out5/1 -> Scope1/3
  Gateway Out6/1 -> Scope1/4
  spead_unpack/5(error) -> Gateway Out6/1, bus_create4/1(in1), [up_spead_error0]
  Counter1/1 -> Gateway Out8/1
  Gateway Out8/1 -> Scope1/5
  pipeline4/1(q) -> digitiser_data_unpack0/1(start64)
  pipeline5/1(q) -> digitiser_data_unpack0/2(data64)
  pipeline6/1(q) -> digitiser_data_unpack0/3(valid64)
  pipeline7/1(q) -> digitiser_data_unpack0/4(eofi)
  pipeline8/1(q) -> digitiser_data_unpack0/5(misci)
  pipeline9/1(q) -> digitiser_data_unpack1/1(start64)
  pipeline10/1(q) -> digitiser_data_unpack1/2(data64)
  pipeline11/1(q) -> digitiser_data_unpack1/3(valid64)
  pipeline12/1(q) -> digitiser_data_unpack1/4(eofi)
  pipeline13/1(q) -> digitiser_data_unpack1/5(misci)
  pipeline14/1(q) -> digitiser_data_unpack2/1(start64)
  pipeline15/1(q) -> digitiser_data_unpack2/2(data64)
  pipeline16/1(q) -> digitiser_data_unpack2/3(valid64)
  pipeline17/1(q) -> digitiser_data_unpack2/4(eofi)
  pipeline18/1(q) -> digitiser_data_unpack2/5(misci)
  pipeline19/1(q) -> digitiser_data_unpack3/1(start64)
  pipeline20/1(q) -> digitiser_data_unpack3/2(data64)
  pipeline21/1(q) -> digitiser_data_unpack3/3(valid64)
  pipeline22/1(q) -> digitiser_data_unpack3/4(eofi)
  pipeline23/1(q) -> digitiser_data_unpack3/5(misci)
